simulink model "flight_simulation"  (R2025b)
settings: Solver=VariableStepAuto  StartTime=0.0  StopTime=10.0  RelTol=1e-3
libraries: aerolibatmos2 x1
settings Model: Creator=user  LastModifiedBy=user

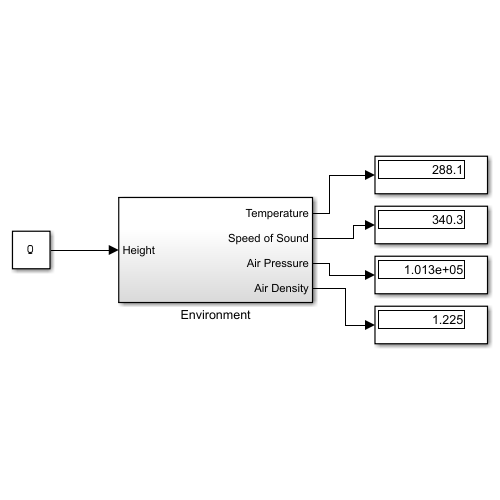
[thumbnail: Simulink's stored preview of the top-level diagram]
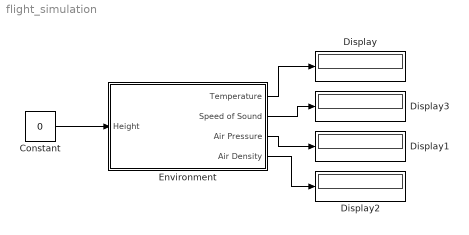
== system flight_simulation ==
  Constant : Constant  Value=0
  Display{,1..3} (4 alike) : Display
  Environment : Subsystem
  wires:
  Constant/1 -> Environment/1(Height)
  Environment/1(Temperature) -> Display/1
  Environment/2(Speed of Sound) -> Display3/1
  Environment/3(Air Pressure) -> Display1/1
  Environment/4(Air Density) -> Display2/1

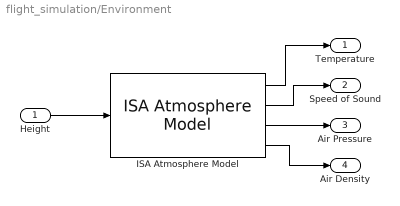
== system flight_simulation/Environment ==
  Height : Inport
  ISA Atmosphere Model : aerolibatmos2/ISA Atmosphere Model  useExtended=off  action=None  custom=off  viscosityOut=off  g=9.80665  gamma=1.4  R=287.0531  L=0.0065  h_trop=11000  h_strat=20000  rho0=1.225  P0=101325  T0=288.15  h0=0  S=110.4  Tref=273.15  muref=1.716e-5
  Temperature : Outport
  Speed of Sound : Outport  Port=2
  Air Pressure : Outport  Port=3
  Air Density : Outport  Port=4
  wires:
  ISA Atmosphere Model/3 -> Air Pressure/1
  ISA Atmosphere Model/4 -> Air Density/1
  ISA Atmosphere Model/1 -> Temperature/1
  ISA Atmosphere Model/2 -> Speed of Sound/1
  Height/1 -> ISA Atmosphere Model/1
